simulink model "component"  (R2018a)
settings: Solver=VariableStepAuto  StartTime=0.0  StopTime=10.0  RelTol=1e-3
settings Model: Creator=Raval  LastModifiedBy=Raval

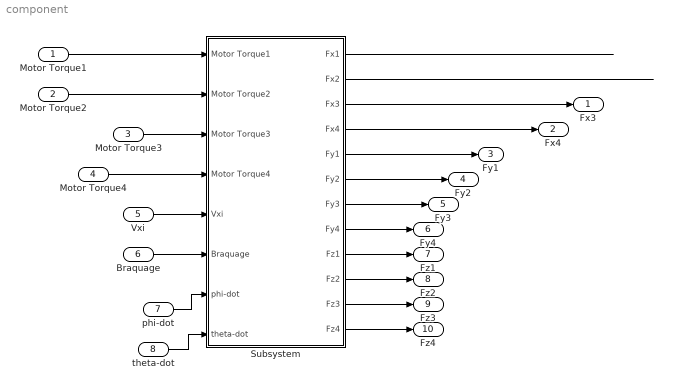
== system component ==
  Motor Torque1 : Inport
  Motor Torque2 : Inport  Port=2
  Motor Torque3 : Inport  Port=3
  Motor Torque4 : Inport  Port=4
  Vxi : Inport  Port=5
  Braquage : Inport  Port=6
  phi-dot : Inport  Port=7
  theta-dot : Inport  Port=8
  Subsystem : Subsystem
  Fx3 : Outport
  Fx4 : Outport  Port=2
  Fy1 : Outport  Port=3
  Fy2 : Outport  Port=4
  Fy3 : Outport  Port=5
  Fy4 : Outport  Port=6
  Fz1 : Outport  Port=7
  Fz2 : Outport  Port=8
  Fz3 : Outport  Port=9
  Fz4 : Outport  Port=10
  wires:
  Subsystem/11(Fz3) -> Fz3/1
  Subsystem/9(Fz1) -> Fz1/1
  Subsystem/12(Fz4) -> Fz4/1
  Subsystem/7(Fy3) -> Fy3/1
  Subsystem/5(Fy1) -> Fy1/1
  Subsystem/10(Fz2) -> Fz2/1
  Subsystem/6(Fy2) -> Fy2/1
  Subsystem/2(Fx2) -> ?
  Subsystem/3(Fx3) -> Fx3/1
  Subsystem/8(Fy4) -> Fy4/1
  theta-dot/1 -> Subsystem/8(theta-dot)
  Subsystem/1(Fx1) -> ?
  Subsystem/4(Fx4) -> Fx4/1
  Vxi/1 -> Subsystem/5(Vxi)
  Braquage/1 -> Subsystem/6(Braquage)
  phi-dot/1 -> Subsystem/7(phi-dot)
  Motor Torque2/1 -> Subsystem/2(Motor Torque2)
  Motor Torque3/1 -> Subsystem/3(Motor Torque3)
  Motor Torque4/1 -> Subsystem/4(Motor Torque4)
  Motor Torque1/1 -> Subsystem/1(Motor Torque1)

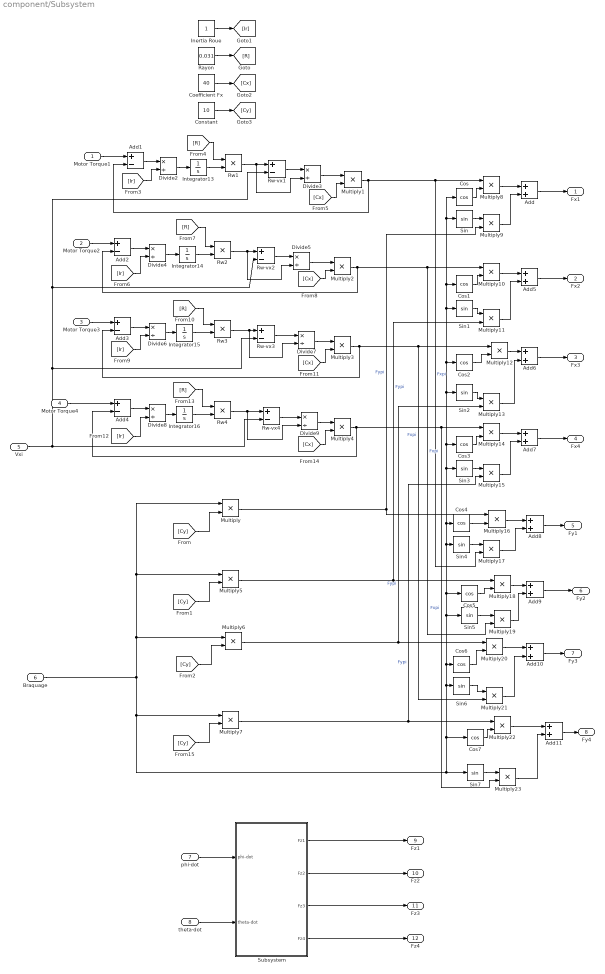
== system component/Subsystem ==
  Motor Torque1 : Inport
  Motor Torque2 : Inport  Port=2
  Motor Torque3 : Inport  Port=3
  Motor Torque4 : Inport  Port=4
  Vxi : Inport  Port=5
  Braquage : Inport  Port=6
  phi-dot : Inport  Port=7
  theta-dot : Inport  Port=8
  Add{,5..11} (8 alike) : Sum
  Add{1..4} (4 alike) : Sum  Inputs=+-
  Coefficient Fx : Constant  Value=40
  Constant : Constant  Value=10
  Cos{,1..7} (8 alike) : Trigonometry  Operator=cos
  Divide{2..9} (8 alike) : Product  Inputs=*/
  Inertia Roue : Constant
  Integrator{13..16} (4 alike) : Integrator
  Multiply{,1..23} (24 alike) : Product
  Rayon : Constant  Value=0.031
  Rw-vx{1..4} (4 alike) : Sum  Inputs=+-
  Rw{1..4} (4 alike) : Product
  Sin{,1..7} (8 alike) : Trigonometry
  Subsystem : Subsystem
  Fx1 : Outport
  Fx2 : Outport  Port=2
  Fx3 : Outport  Port=3
  Fx4 : Outport  Port=4
  Fy1 : Outport  Port=5
  Fy2 : Outport  Port=6
  Fy3 : Outport  Port=7
  Fy4 : Outport  Port=8
  Fz1 : Outport  Port=9
  Fz2 : Outport  Port=10
  Fz3 : Outport  Port=11
  Fz4 : Outport  Port=12
  wires:
  Multiply7/1 -> Multiply22/1, Multiply15/2  "Fypi"
  Rw2/1 -> Divide5/2, Rw-vx2/1
  Add1/1 -> Divide2/1
  Constant/1 -> [Cy]
  Motor Torque1/1 -> Add1/1
  Sin5/1 -> Multiply19/1
  Braquage/1 -> Multiply6/1, Multiply5/1, Multiply/1, Cos7/1, Cos6/1, Cos2/1, Cos1/1, Cos/1, Sin/1, Sin1/1, Sin2/1, Cos3/1, Sin3/1, Cos4/1, Sin4/1, Cos5/1, Sin5/1, Sin6/1, Sin7/1, Multiply7/1
  Add6/1 -> Fx3/1
  Multiply11/1 -> Add5/2
  Sin/1 -> Multiply9/1
  Multiply12/1 -> Add6/1
  Multiply23/1 -> Add11/2
  Rw-vx1/1 -> Divide3/1
  Multiply13/1 -> Add6/2
  [Cy] -> Multiply/2
  Sin1/1 -> Multiply11/1
  Vxi/1 -> Rw-vx4/2, Rw-vx2/2, Rw-vx1/2, Rw-vx3/2
  [Ir] -> Divide6/2
  Multiply14/1 -> Add7/1
  [Ir] -> Divide8/2
  Multiply15/1 -> Add7/2
  [Cy] -> Multiply6/2
  Add11/1 -> Fy4/1
  Multiply10/1 -> Add5/1
  Add10/1 -> Fy3/1
  Multiply8/1 -> Add/1
  Integrator16/1 -> Rw4/2
  Divide3/1 -> Multiply1/1
  Multiply4/1 -> Add4/2, Multiply23/2, Multiply14/1  "Fxpi"
  Sin6/1 -> Multiply21/1
  Divide5/1 -> Multiply2/1
  Cos/1 -> Multiply8/2
  Divide2/1 -> Integrator13/1
  Divide8/1 -> Integrator16/1
  Rw3/1 -> Divide7/2, Rw-vx3/1
  [Ir] -> Divide2/2
  Rw1/1 -> Divide3/2, Rw-vx1/1
  Rw4/1 -> Divide9/2, Rw-vx4/1
  Add7/1 -> Fx4/1
  Divide7/1 -> Multiply3/1
  [Cy] -> Multiply5/2
  Multiply1/1 -> Multiply8/1, Multiply17/2, Add1/2  "Fxpi"
  [Cy] -> Multiply7/2
  Motor Torque2/1 -> Add2/1
  Multiply/1 -> Multiply9/2, Multiply16/1  "Fypi"
  Multiply6/1 -> Multiply20/1, Multiply13/2  "Fypi"
  Motor Torque3/1 -> Add3/1
  Multiply20/1 -> Add10/1
  Multiply17/1 -> Add8/2
  Integrator14/1 -> Rw2/2
  [Cx] -> Multiply1/2
  Coefficient Fx/1 -> [Cx]
  Rayon/1 -> [R]
  Multiply21/1 -> Add10/2
  [Cx] -> Multiply2/2
  Multiply2/1 -> Add2/2, Multiply19/2, Multiply10/1  "Fxpi"
  Add3/1 -> Divide6/1
  [R] -> Rw1/1
  [Cx] -> Multiply4/2
  [Cx] -> Multiply3/2
  Integrator15/1 -> Rw3/2
  [R] -> Rw3/1
  Divide6/1 -> Integrator15/1
  Rw-vx3/1 -> Divide7/1
  Add2/1 -> Divide4/1
  Divide9/1 -> Multiply4/1
  [R] -> Rw4/1
  Multiply9/1 -> Add/2
  Multiply3/1 -> Add3/2, Multiply21/2, Multiply12/1  "Fxpi"
  Motor Torque4/1 -> Add4/1
  Cos1/1 -> Multiply10/2
  Sin3/1 -> Multiply15/1
  Cos2/1 -> Multiply12/2
  Add5/1 -> Fx2/1
  Cos4/1 -> Multiply16/2
  Sin4/1 -> Multiply17/1
  Multiply18/1 -> Add9/1
  Add8/1 -> Fy1/1
  Add9/1 -> Fy2/1
  Multiply16/1 -> Add8/1
  Add4/1 -> Divide8/1
  Multiply19/1 -> Add9/2
  [Ir] -> Divide4/2
  Cos5/1 -> Multiply18/2
  Multiply22/1 -> Add11/1
  Multiply5/1 -> Multiply18/1, Multiply11/2  "Fypi"
  Cos6/1 -> Multiply20/2
  Rw-vx4/1 -> Divide9/1
  Divide4/1 -> Integrator14/1
  Inertia Roue/1 -> [Ir]
  Cos7/1 -> Multiply22/2
  Integrator13/1 -> Rw1/2
  Add/1 -> Fx1/1
  Rw-vx2/1 -> Divide5/1
  Sin7/1 -> Multiply23/1
  Sin2/1 -> Multiply13/1
  [R] -> Rw2/1
  Cos3/1 -> Multiply14/2
  phi-dot/1 -> Subsystem/1(phi-dot)
  theta-dot/1 -> Subsystem/2(theta-dot)
  Subsystem/1(Fz1) -> Fz1/1
  Subsystem/2(Fz2) -> Fz2/1
  Subsystem/3(Fz3) -> Fz3/1
  Subsystem/4(Fz4) -> Fz4/1

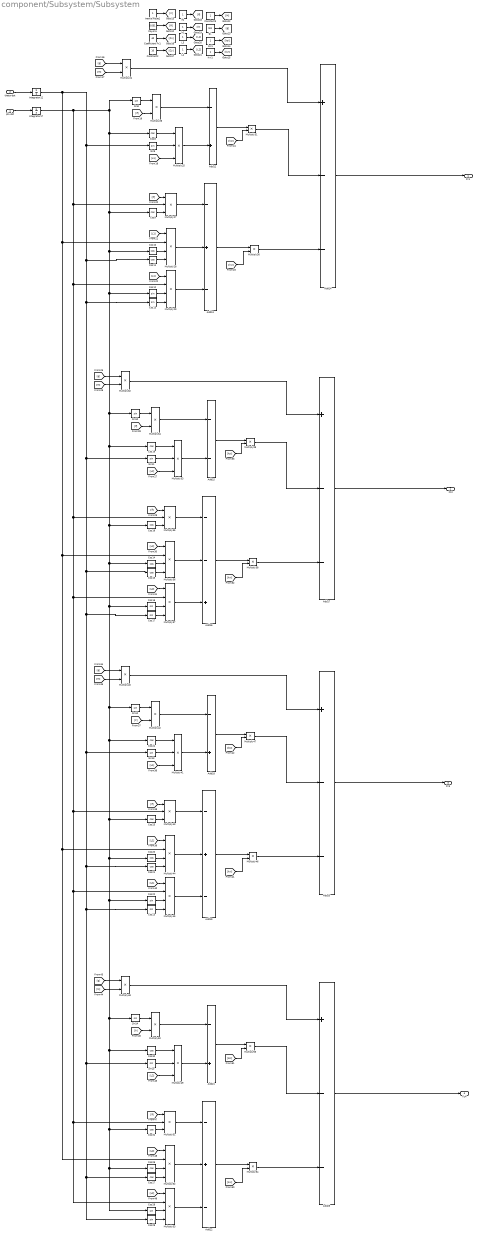
== system component/Subsystem/Subsystem ==
  phi-dot : Inport
  theta-dot : Inport  Port=2
  Add12 : Sum  Inputs=-+
  Add13 : Sum  Inputs=-+-
  Add{14,17,20,23} (4 alike) : Sum  Inputs=+--
  Add15 : Sum  Inputs=--
  Add16 : Sum  Inputs=--+
  Add18 : Sum  Inputs=-+
  Add19 : Sum  Inputs=-+-
  Add21 : Sum  Inputs=-+
  Add22 : Sum  Inputs=-+-
  Coefficient Fx1 : Constant  Value=40
  Constant2 : Constant  Value=10
  Constant3 : Constant
  Cos{8..11,14..15,18..21,24..27,30..31} (16 alike) : Trigonometry  Operator=cos
  Cos{12..13,16..17,22..23,28..29} (8 alike) : Trigonometry
  Inertia Roue1 : Constant
  Integrator12 : Integrator
  Integrator17 : Integrator
  Kvi1 : Constant
  L3 : Constant
  L4 : Constant
  Multiply{24,26,30..32,34,38..40,42,46..48,50,54..55} (16 alike) : Product
  Multiply{25,27,33,35,41,43,49,51} (8 alike) : Product  Inputs=3
  Multiply{28..29,36..37,44..45,52..53} (8 alike) : Product  Inputs=4
  Rayon1 : Constant  Value=0.031
  Sin{8..15} (8 alike) : Trigonometry
  g1 : Constant  Value=9.8
  ksi1 : Constant
  lf1 : Constant
  lr1 : Constant
  Fz1 : Outport
  Fz2 : Outport  Port=2
  Fz3 : Outport  Port=3
  Fz4 : Outport  Port=4
  wires:
  Cos17/1 -> Multiply37/4
  Coefficient Fx1/1 -> [Cx]
  ksi1/1 -> [ksi]
  Constant2/1 -> [Cy]
  Sin10/1 -> Multiply34/1
  lf1/1 -> [lf]
  Multiply37/1 -> Add16/3
  Multiply38/1 -> Add17/3
  Add22/1 -> Multiply54/1
  Add20/1 -> Fz3/1
  [L1] -> Multiply45/1
  Multiply45/1 -> Add19/3
  g1/1 -> [g]
  Sin8/1 -> Multiply26/1
  lr1/1 -> [lr]
  Add14/1 -> Fz1/1
  Multiply25/1 -> Add12/2
  Multiply47/1 -> Add20/2
  Kvi1/1 -> [kvi]
  [L2] -> Multiply49/3
  [M] -> Multiply24/2
  Constant3/1 -> [M]
  Multiply33/1 -> Add15/2
  [lf] -> Multiply51/1
  [kvi] -> Multiply38/2
  L3/1 -> [L1]
  [L1] -> Multiply29/1
  Multiply36/1 -> Add16/2
  Multiply52/1 -> Add22/2
  Cos19/1 -> Multiply35/3
  Rayon1/1 -> [R]
  Inertia Roue1/1 -> [Ir]
  [lf] -> Multiply34/2
  Add17/1 -> Fz2/1
  L4/1 -> [L2]
  phi-dot/1 -> Integrator17/1
  Sin13/1 -> Multiply41/2
  Multiply31/1 -> Add14/2
  Cos22/1 -> Multiply45/3
  Integrator17/1 -> Multiply53/2, Multiply51/2, Multiply45/2, Multiply43/2, Multiply37/2, Multiply35/2, Multiply29/2, Multiply27/2, Cos9/1, Cos28/1, Cos26/1, Cos31/1, Cos30/1, Sin14/1, Cos22/1, Cos20/1, Cos25/1, Cos24/1, Sin12/1, Cos16/1, Cos14/1, Cos19/1, Cos18/1, Sin10/1, Cos12/1, Cos10/1, Cos8/1, Sin8/1
  Cos14/1 -> Multiply36/3
  [L2] -> Multiply33/3
  Integrator12/1 -> Multiply52/2, Multiply44/2, Multiply36/2, Multiply28/2, Cos11/1, Cos13/1, Cos15/1, Cos17/1, Cos21/1, Cos23/1, Cos29/1, Cos27/1, Sin15/1, Sin13/1, Sin11/1, Sin9/1
  Multiply26/1 -> Add12/1
  Cos11/1 -> Multiply28/4
  [kvi] -> Multiply30/2
  Add21/1 -> Multiply55/1
  [g] -> Multiply24/1
  Add13/1 -> Multiply30/1
  Cos10/1 -> Multiply28/3
  Cos20/1 -> Multiply44/3
  theta-dot/1 -> Integrator12/1
  Cos8/1 -> Multiply25/1
  Multiply44/1 -> Add19/2
  Add23/1 -> Fz4/1
  [L1] -> Multiply44/1
  Sin9/1 -> Multiply25/2
  Cos18/1 -> Multiply33/1
  [L2] -> Multiply53/1
  [L1] -> Multiply28/1
  Multiply43/1 -> Add19/1
  Cos23/1 -> Multiply45/4
  Add15/1 -> Multiply39/1
  [lf] -> Multiply27/1
  [M] -> Multiply40/2
  Multiply35/1 -> Add16/1
  [g] -> Multiply32/1
  Multiply24/1 -> Add14/1
  Add19/1 -> Multiply46/1
  [L2] -> Multiply36/1
  Cos26/1 -> Multiply52/3
  Multiply27/1 -> Add13/1
  [lr] -> Multiply50/2
  [lf] -> Multiply43/1
  [L1] -> Multiply41/3
  [g] -> Multiply40/1
  Cos28/1 -> Multiply53/3
  [kvi] -> Multiply54/2
  Sin11/1 -> Multiply33/2
  Cos25/1 -> Multiply43/3
  Multiply55/1 -> Add23/2
  Multiply28/1 -> Add13/2
  [kvi] -> Multiply46/2
  Add12/1 -> Multiply31/1
  Cos31/1 -> Multiply51/3
  Cos21/1 -> Multiply44/4
  [M] -> Multiply48/2
  [M] -> Multiply32/2
  Sin15/1 -> Multiply49/2
  Cos16/1 -> Multiply37/3
  [ksi] -> Multiply31/2
  Multiply42/1 -> Add18/1
  Multiply54/1 -> Add23/3
  Multiply30/1 -> Add14/3
  Multiply41/1 -> Add18/2
  Multiply48/1 -> Add23/1
  [lf] -> Multiply26/2
  [L2] -> Multiply37/1
  Multiply29/1 -> Add13/3
  Multiply51/1 -> Add22/1
  [ksi] -> Multiply39/2
  [ksi] -> Multiply47/2
  Multiply40/1 -> Add20/1
  [lr] -> Multiply42/2
  Multiply39/1 -> Add17/2
  Multiply34/1 -> Add15/1
  Cos30/1 -> Multiply49/1
  Cos9/1 -> Multiply27/3
  [g] -> Multiply48/1
  [lf] -> Multiply35/1
  Multiply32/1 -> Add17/1
  Cos15/1 -> Multiply36/4
  Cos13/1 -> Multiply29/4
  [ksi] -> Multiply55/2
  Cos27/1 -> Multiply52/4
  Cos12/1 -> Multiply29/3
  Cos24/1 -> Multiply41/1
  Sin12/1 -> Multiply42/1
  Multiply53/1 -> Add22/3
  Multiply49/1 -> Add21/2
  Add18/1 -> Multiply47/1
  [L2] -> Multiply52/1
  Add16/1 -> Multiply38/1
  Cos29/1 -> Multiply53/4
  Sin14/1 -> Multiply50/1
  [L1] -> Multiply25/3
  Multiply46/1 -> Add20/3
  Multiply50/1 -> Add21/1
